simulink model "DR_telemedicine"  (R2026a)
settings: Solver=VariableStepAuto  StopTime=250
settings Model: Creator=hp  LastModifiedBy=hp

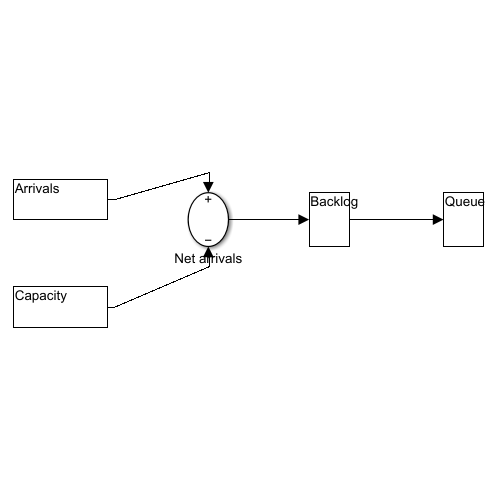
[thumbnail: Simulink's stored preview of the top-level diagram]
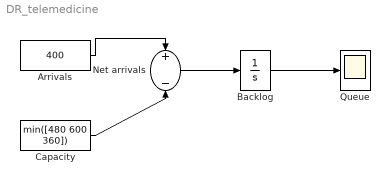
== system DR_telemedicine ==
  Arrivals : Constant  Value=400
  Backlog : Integrator  LimitOutput=on  LowerSaturationLimit=0
  Capacity : Constant  Value=min([480 600 360])
  Net arrivals : Sum  Inputs=+-
  Queue : Scope
  wires:
  Arrivals/1 -> Net arrivals/1
  Capacity/1 -> Net arrivals/2
  Net arrivals/1 -> Backlog/1
  Backlog/1 -> Queue/1
